simulink model "statefdbk"  (R2019b)
settings: Solver=VariableStepAuto  StartTime=0.0  StopTime=T  RelTol=1e-3
values from neighbouring files (symbols this model uses):
  A = A*(v_phi(k,i)*s^i)    [Roberts_Q_design.m]    (also in main_fmincon.m = []; rocket_model.m = [0,1,0,0,0,0; ss_model.mat = [0  0; 1  0]; verif.m = [0,1;0,0])
  B = B*(s-alpha(i))    [Roberts_Q_design.m]    (also in controller_design.m = B*C(2); main_yp_fminunc.m = B*C(2); rocket_controllerdesign.m = B*C(2); rocket_controllerdesign_z.m = B*C(2))
  C = [0,1]    [controller_design.m]    (also in main_yp_fminunc.m; rocket_controllerdesign.m; rocket_controllerdesign_z.m; rocket_model.m = eye(6))
  K = minreal(Q/(1+Q*P))    [cost.m]    (also in cost_LQ.m = tf((conv(denQ{1},numK0{1})+conv(numQ{1},den_sys{1})),(conv(d; cost_con.m = tf((conv(denQ{1},numK0{1})+conv(numQ{1},den_sys{1})),(conv(d; cost_disturb.m = tf((conv(denQ{1},numK0{1})+conv(numQ{1},den_sys{1})),(conv(d; fminunc_LQ.m = tf((conv(denQ{1},numK0{1})+conv(numQ{1},den_sys{1})),(conv(d)
  Nbar = rscale(A,B,C,D,K)    [controller_design.m]    (also in rocket_controllerdesign.m; rocket_controllerdesign_z.m; sim_controller_design.m = -inv(C*inv(A-B*K)*B))
undefined symbols (not defined in the file or in its folder): C_sim
settings Model: Creator=alice  LastModifiedBy=bia
settings SFSimCC: CustomCodeUndefinedFunction=UseInterfaceOnly

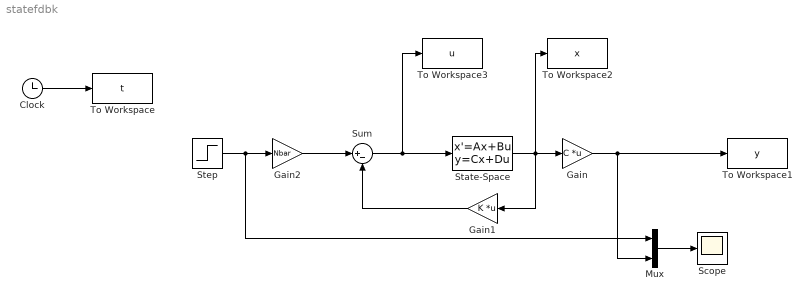
== system statefdbk ==
  Clock : Clock
  Gain : Gain  Gain=C  Multiplication=Matrix(K*u)
  Gain1 : Gain  Gain=K  Multiplication=Matrix(K*u)
  Gain2 : Gain  Gain=Nbar
  Mux : Mux  Inputs=2
  Scope : Scope
  State-Space : StateSpace  A=A  B=B  C=C_sim  D=[0;0]  InitialCondition=0
  Step : Step  SampleTime=0
  Sum : Sum  Inputs=|+-
  To Workspace : ToWorkspace  VariableName=t  SampleTime=-1
  To Workspace1 : ToWorkspace  VariableName=y  SampleTime=-1
  To Workspace2 : ToWorkspace  VariableName=x  SampleTime=-1
  To Workspace3 : ToWorkspace  VariableName=u  SampleTime=-1
  wires:
  Step/1 -> Mux/1, Gain2/1
  Gain2/1 -> Sum/1
  Sum/1 -> To Workspace3/1, State-Space/1
  Gain1/1 -> Sum/2
  State-Space/1 -> To Workspace2/1, Gain1/1, Gain/1
  Gain/1 -> Mux/2, To Workspace1/1
  Mux/1 -> Scope/1
  Clock/1 -> To Workspace/1
